simulink model "UDP_1"  (R2013b)
settings: Solver=ode45  StartTime=0.0  StopTime=1000  MaxStep=0.01  MinStep=0.01  RelTol=1e-3
libraries: xpclib x1, dspnetwork x1
settings Model: Creator=lankuohsing  LastModifiedBy=lankuohsing
settings SolverCC: InitialStep=0.01

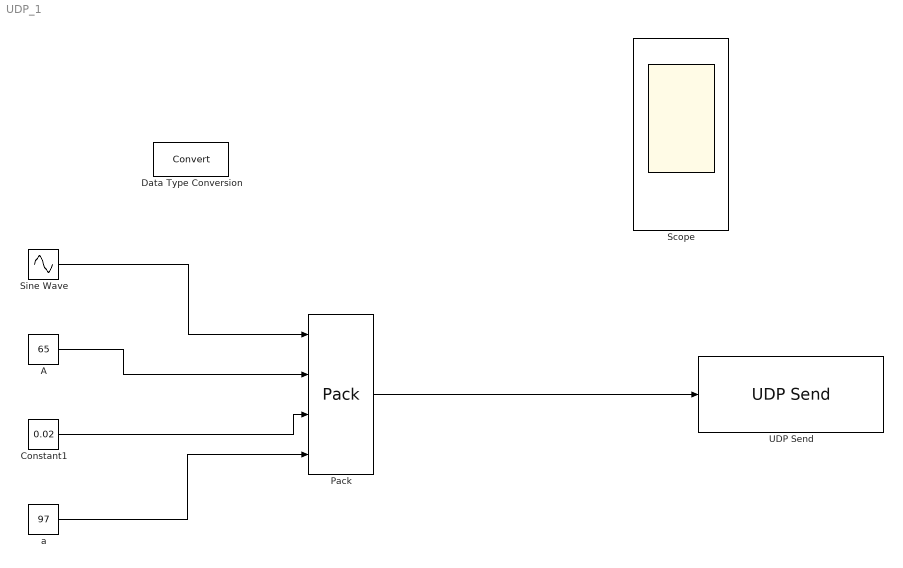
== system UDP_1 ==
  A : Constant  Value=65
  Constant1 : Constant  Value=0.02
  Data Type Conversion : DataTypeConversion
  Pack : xpclib/UDP/Pack  datatypes={'double','double','double','double'}  byteAlign=1
  Scope : Scope  NumInputPorts=4
      settings: YMin=-5~-5~-5~-5  YMax=5~5~5~5
  Sine Wave : Sin  SampleTime=0
  UDP Send : dspnetwork/UDP Send  remoteURL='255.255.255.255'  remotePort=9090  localURL='0.0.0.0'  localPortSource=Specify via dialog  localPort=9091  sampletime=-1  blockPlatform=HOST  separateLengthPort=0
  a : Constant  Value=97
  wires:
  Pack/1 -> UDP Send/1
  Sine Wave/1 -> Pack/1
  A/1 -> Pack/2
  Constant1/1 -> Pack/3
  a/1 -> Pack/4
